simulink model "PrevThrustTestingNew"  (R2018b)
settings: Solver=ode4  StartTime=0.0  StopTime=34560000  FixedStep=10  RelTol=1e-3
InitFcn:
  | % Enter your data here
  | 
  | y10 = 152213668;
  | y20 = 0;
  | y30 = 0;
  | y40 = 0;
  | y50 = 34.5845;
  | y60 = 0;
  | y70 = 9700;
settings Model: Creator=jhemi.1  LastModifiedBy=Vitamin-Z
settings DebuggingCC: LibraryContextMissingDiagnostic=none
settings SFSimCC: SimUseLocalCustomCode=off
settings RTWCC: RTWUseLocalCustomCode=off
settings CodeAppCC: StateflowObjectComments=on

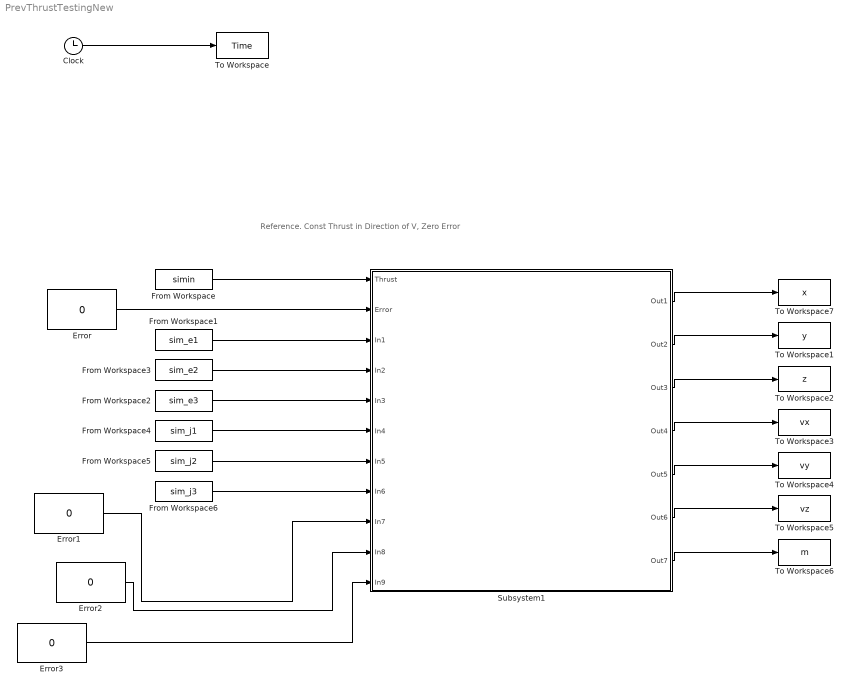
== system PrevThrustTestingNew ==
  note: Reference. Const Thrust in Direction of V, Zero Error
  Clock : Clock
  Error{,1..3} (4 alike) : Constant  Value=0
  From Workspace : FromWorkspace  VariableName=simin  SampleTime=0
  From Workspace1 : FromWorkspace  VariableName=sim_e1  SampleTime=0
  From Workspace2 : FromWorkspace  VariableName=sim_e3  SampleTime=0
  From Workspace3 : FromWorkspace  VariableName=sim_e2  SampleTime=0
  From Workspace4 : FromWorkspace  VariableName=sim_j1  SampleTime=0
  From Workspace5 : FromWorkspace  VariableName=sim_j2  SampleTime=0
  From Workspace6 : FromWorkspace  VariableName=sim_j3  SampleTime=0
  Subsystem1 : Subsystem
  To Workspace : ToWorkspace  VariableName=Time  SampleTime=-1
  To Workspace1 : ToWorkspace  VariableName=y  SampleTime=-1
  To Workspace2 : ToWorkspace  VariableName=z  SampleTime=-1
  To Workspace3 : ToWorkspace  VariableName=vx  SampleTime=-1
  To Workspace4 : ToWorkspace  VariableName=vy  SampleTime=-1
  To Workspace5 : ToWorkspace  VariableName=vz  SampleTime=-1
  To Workspace6 : ToWorkspace  VariableName=m  SampleTime=-1
  To Workspace7 : ToWorkspace  VariableName=x  SampleTime=-1
  wires:
  Clock/1 -> To Workspace/1
  Subsystem1/1(Out1) -> To Workspace7/1
  Subsystem1/2(Out2) -> To Workspace1/1
  Subsystem1/3(Out3) -> To Workspace2/1
  Subsystem1/4(Out4) -> To Workspace3/1
  Subsystem1/5(Out5) -> To Workspace4/1
  Subsystem1/6(Out6) -> To Workspace5/1
  Subsystem1/7(Out7) -> To Workspace6/1
  Error/1 -> Subsystem1/2(Error)
  From Workspace/1 -> Subsystem1/1(Thrust)
  From Workspace1/1 -> Subsystem1/3(In1)
  From Workspace3/1 -> Subsystem1/4(In2)
  From Workspace2/1 -> Subsystem1/5(In3)
  From Workspace4/1 -> Subsystem1/6(In4)
  From Workspace5/1 -> Subsystem1/7(In5)
  From Workspace6/1 -> Subsystem1/8(In6)
  Error1/1 -> Subsystem1/9(In7)
  Error2/1 -> Subsystem1/10(In8)
  Error3/1 -> Subsystem1/11(In9)

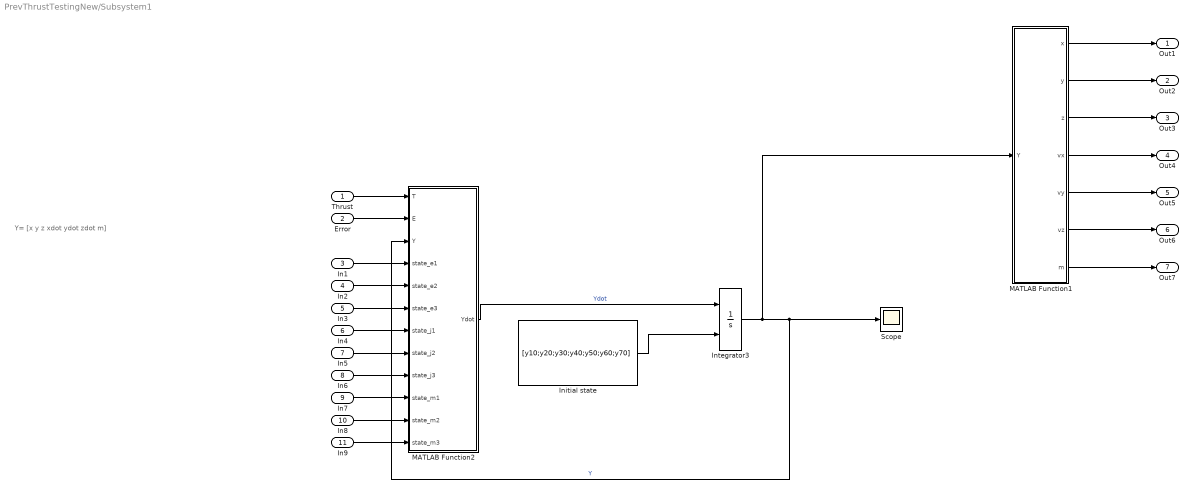
== system PrevThrustTestingNew/Subsystem1 ==
  note: Y= [x
      | y
      | z
      | xdot
      | ydot
      | zdot
      | m]
  Thrust : Inport
  Error : Inport  Port=2
  In1 : Inport  Port=3
  In2 : Inport  Port=4
  In3 : Inport  Port=5
  In4 : Inport  Port=6
  In5 : Inport  Port=7
  In6 : Inport  Port=8
  In7 : Inport  Port=9
  In8 : Inport  Port=10
  In9 : Inport  Port=11
  Initial state : Constant  Value=[y10;y20;y30;y40;y50;y60;y70]
  Integrator3 : Integrator  InitialConditionSource=external
  MATLAB Function1 : MATLAB Function  TreatAsAtomicUnit=on
  MATLAB Function2 : MATLAB Function  TreatAsAtomicUnit=on
  Scope : Scope
  Out1 : Outport
  Out2 : Outport  Port=2
  Out3 : Outport  Port=3
  Out4 : Outport  Port=4
  Out5 : Outport  Port=5
  Out6 : Outport  Port=6
  Out7 : Outport  Port=7
  wires:
  MATLAB Function1/1(x) -> Out1/1
  MATLAB Function2/1(Ydot) -> Integrator3/1  "Ydot"
  MATLAB Function1/5(vy) -> Out5/1
  Thrust/1 -> MATLAB Function2/1(T)
  MATLAB Function1/4(vx) -> Out4/1
  Integrator3/1 -> MATLAB Function1/1(Y), MATLAB Function2/3(Y), Scope/1  "Y"
  MATLAB Function1/6(vz) -> Out6/1
  MATLAB Function1/3(z) -> Out3/1
  MATLAB Function1/2(y) -> Out2/1
  Initial state/1 -> Integrator3/2
  MATLAB Function1/7(m) -> Out7/1
  Error/1 -> MATLAB Function2/2(E)
  In1/1 -> MATLAB Function2/4(state_e1)
  In2/1 -> MATLAB Function2/5(state_e2)
  In3/1 -> MATLAB Function2/6(state_e3)
  In4/1 -> MATLAB Function2/7(state_j1)
  In5/1 -> MATLAB Function2/8(state_j2)
  In6/1 -> MATLAB Function2/9(state_j3)
  In7/1 -> MATLAB Function2/10(state_m1)
  In8/1 -> MATLAB Function2/11(state_m2)
  In9/1 -> MATLAB Function2/12(state_m3)

== matlab function PrevThrustTestingNew/Subsystem1/MATLAB Function1 ==
  data: x output; y output; z output; vx output; vy output; vz output; Y input; m output
function [x,y,z,vx,vy,vz,m] = fcn(Y)
% This function does ......,.
%
% constants
 

% reading the OED variable from Y
x = Y(1);  % x
y = Y(2);  % y
z = Y(3);  % z
vx = Y(4);  % xdot
vy = Y(5);  % ydot
vz = Y(6);  % zdot
m  = Y(7);  % m



 
% end of function

== matlab function PrevThrustTestingNew/Subsystem1/MATLAB Function2 ==
  data: T input; E input; Y input; Ydot output; state_e1 input; state_e2 input; state_e3 input; state_j1 input; state_j2 input; state_j3 input; state_m1 input; state_m2 input; state_m3 input
function Ydot = fcn(T,E,Y,state_e1,state_e2,state_e3,state_j1,state_j2,state_j3,state_m1,state_m2,state_m3)
% This function does ......,.
% T = thrust [N]
% E = error/noise

% constants
Isp = 850;
g0 = 9.81*10^-3;
G      = 6.67408*10^-20;    % Gravitational Constant [km^3/kgs^2]

m_e    = 5.9723*10^24;      % Mass of Earth [kg]
m_m    = 641.9*10^21;       % Mass of Mars [kg]
m_j    = 1.898*10^27;       % Mass of Jupiter [kg]
m_s    = 1.989*10^30;       % Mass of Sun [kg]

u_s    = G*m_s;             % mu Sun [km^3/s^2]
u_e    = G*m_e;             % mu Earth [km^3/s^2]
u_m    = G*m_m;             % mu Mars [km^3/s^2]
u_j    = G*m_j;             % mu Jupiter [km^3/s^2]

% reading the OED variable from Y
y1 = Y(1);  % x
y2 = Y(2);  % y
y3 = Y(3);  % z
y4 = Y(4);  % xdot
y5 = Y(5);  % ydot
y6 = Y(6);  % zdot
m  = Y(7);  % m

% Computing velocity, position 
V = sqrt(y4^2+y5^2+y6^2); % velocity
r = sqrt(y1^2+y2^2+y3^2); % position

r_earth = zeros(1,3);
r_earth(1) = y1 - state_e1;
r_earth(2) = y2 - state_e2;
r_earth(3) = y3 - state_e3;
r_emag = norm(r_earth);

r_jupiter = zeros(1,3);
r_jupiter(1) = y1 - state_j1;
r_jupiter(2) = y2 - state_j2;
r_jupiter(3) = y3 - state_j3;
r_jmag = norm(r_jupiter);

r_mars = zeros(1,3);
r_mars(1) = y1 - state_m1;
r_mars(2) = y2 - state_m2;
r_mars(3) = y3 - state_m3;
r_mmag = norm(r_mars);

%
% Computing Ydot (ODE implementation)
Ydot = [y4;
        y5;
        y6;
       -u_s*y1/r^3-u_e*r_earth(1)/r_emag^3-u_j*r_jupiter(1)/r_jmag^3-u_m*r_mars(1)/r_mmag^3+T/m*y4/V+E;   
       -u_s*y2/r^3-u_e*r_earth(2)/r_emag^3-u_j*r_jupiter(2)/r_jmag^3-u_m*r_mars(2)/r_mmag^3+T/m*y5/V+E;
       -u_s*y3/r^3-u_e*r_earth(3)/r_emag^3-u_j*r_jupiter(3)/r_jmag^3-u_m*r_mars(3)/r_mmag^3+T/m*y6/V+E;
       -abs(T)/(Isp*g0)
       ];
% End of function.
